simulink model "VTOL_RESPONSE_SIMULINK"  (R2024b)
settings: Solver=FixedStepDiscrete  StartTime=0.0  StopTime=1.5  FixedStep=dt_sim  RelTol=1e-3
InitFcn:
  | if evalin('base','exist(''sim_model'',''var'')') == 0; flap_model_override='disk'; RUN_RESPONSE_SIMULINK_SETUP; end
values from neighbouring files (symbols this model uses):
  rotor_state0 = zeros(n_rotors * response_rotor_state_size, 1)    [RUN_RESPONSE_SIMULINK_SETUP.m]
  rotor_tilt_angle_deg = trim_rotor_tilt_angle_deg(:)    [RUN_RESPONSE_SIMULINK_SETUP.m]
  x0 = trim_results.response.state_history(1,:).'    [RUN_RESPONSE_SIMULINK_SETUP.m]
undefined symbols (not defined in the file or in its folder): control_delta, dt_sim, fixed_control_delta
settings Model: Creator=yuany  LastModifiedBy=yuany

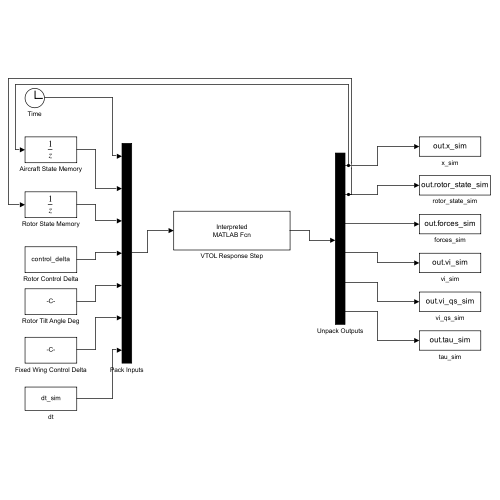
[thumbnail: Simulink's stored preview of the top-level diagram]
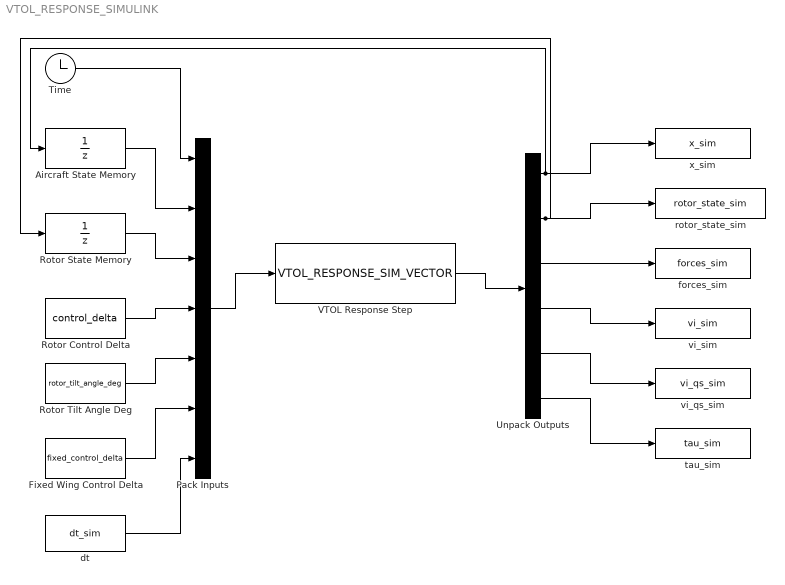
== system VTOL_RESPONSE_SIMULINK ==
  Aircraft State Memory : UnitDelay  InitialCondition=x0  SampleTime=dt_sim  HasFrameUpgradeWarning=on
  Fixed Wing Control Delta : Constant  Value=fixed_control_delta  SampleTime=dt_sim
  Pack Inputs : Mux  Inputs=7
  Rotor Control Delta : Constant  Value=control_delta  SampleTime=dt_sim
  Rotor State Memory : UnitDelay  InitialCondition=rotor_state0  SampleTime=dt_sim  HasFrameUpgradeWarning=on
  Rotor Tilt Angle Deg : Constant  Value=rotor_tilt_angle_deg  SampleTime=dt_sim
  Time : Clock
  Unpack Outputs : Demux  Outputs=[12 42 6 6 6 6]
  VTOL Response Step : MATLABFcn  MATLABFcn=VTOL_RESPONSE_SIM_VECTOR  OutputDimensions=78  SampleTime=dt_sim
  dt : Constant  Value=dt_sim  SampleTime=dt_sim
  forces_sim : ToWorkspace  VariableName=forces_sim  SaveFormat=Structure With Time  SampleTime=-1
  rotor_state_sim : ToWorkspace  VariableName=rotor_state_sim  SaveFormat=Structure With Time  SampleTime=-1
  tau_sim : ToWorkspace  VariableName=tau_sim  SaveFormat=Structure With Time  SampleTime=-1
  vi_qs_sim : ToWorkspace  VariableName=vi_qs_sim  SaveFormat=Structure With Time  SampleTime=-1
  vi_sim : ToWorkspace  VariableName=vi_sim  SaveFormat=Structure With Time  SampleTime=-1
  x_sim : ToWorkspace  VariableName=x_sim  SaveFormat=Structure With Time  SampleTime=-1
  wires:
  Time/1 -> Pack Inputs/1
  Aircraft State Memory/1 -> Pack Inputs/2
  Rotor State Memory/1 -> Pack Inputs/3
  Rotor Control Delta/1 -> Pack Inputs/4
  Rotor Tilt Angle Deg/1 -> Pack Inputs/5
  Fixed Wing Control Delta/1 -> Pack Inputs/6
  dt/1 -> Pack Inputs/7
  Pack Inputs/1 -> VTOL Response Step/1
  VTOL Response Step/1 -> Unpack Outputs/1
  Unpack Outputs/1 -> Aircraft State Memory/1, x_sim/1
  Unpack Outputs/2 -> Rotor State Memory/1, rotor_state_sim/1
  Unpack Outputs/3 -> forces_sim/1
  Unpack Outputs/4 -> vi_sim/1
  Unpack Outputs/5 -> vi_qs_sim/1
  Unpack Outputs/6 -> tau_sim/1
